simulink model "sim_SIL_code_algorithm"  (R2023a)
settings: Solver=FixedStepAuto  StartTime=0.0  StopTime=Inf  FixedStep=0.01  RelTol=1e-3
model workspace (MAT data in the model file):
  Fe = 0.02
  J = 0.01
  Ke = 0.75
  Kt = 0.75
  L = 1.1
  R = 5.2
libraries: sldrtlib x1
settings Model: Creator=Tu  LastModifiedBy=Tu

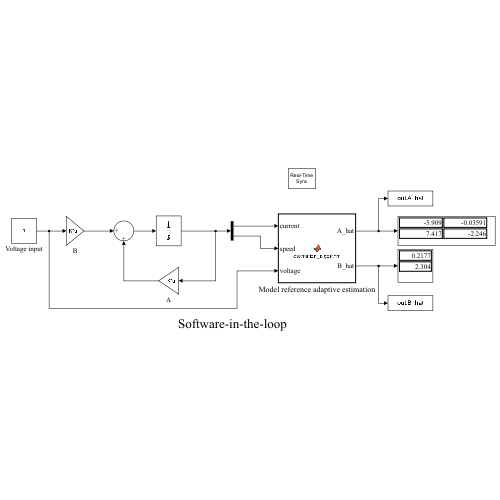
[thumbnail: Simulink's stored preview of the top-level diagram]
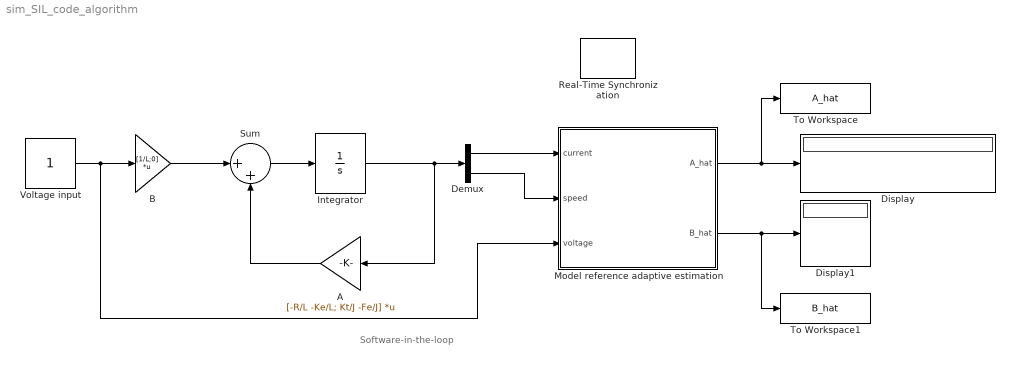
== system sim_SIL_code_algorithm ==
  note: Software-in-the-loop
  A : Gain  Gain=[-R/L -Ke/L; Kt/J -Fe/J]  Multiplication=Matrix(K*u)
  B : Gain  Gain=[1/L;0]  Multiplication=Matrix(K*u)
  Demux : Demux  Outputs=2
  Display : Display
  Display1 : Display
  Integrator : Integrator
  Model reference adaptive estimation : MATLAB Function  TreatAsAtomicUnit=on  SystemSampleTime=0.01
  Real-Time Synchronization : sldrtlib/Real-Time Synchronization  SampleTime=0.01  MaxMissedTicks=100000  ShowMissedTicks=off  YieldWhenWaiting=off
  Sum : Sum  Inputs=|++
  To Workspace : ToWorkspace  VariableName=A_hat  SampleTime=-1
      settings: Save2DSignal=2-D array (concatenate along first dimension)
  To Workspace1 : ToWorkspace  VariableName=B_hat  SampleTime=-1
      settings: Save2DSignal=2-D array (concatenate along first dimension)
  Voltage input : Constant
  wires:
  Sum/1 -> Integrator/1
  Voltage input/1 -> B/1, Model reference adaptive estimation/3(voltage)
  B/1 -> Sum/1
  A/1 -> Sum/2
  Integrator/1 -> A/1, Demux/1
  Demux/2 -> Model reference adaptive estimation/2(speed)
  Demux/1 -> Model reference adaptive estimation/1(current)
  Model reference adaptive estimation/2(B_hat) -> To Workspace1/1, Display1/1
  Model reference adaptive estimation/1(A_hat) -> To Workspace/1, Display/1

== matlab function sim_SIL_code_algorithm/Model reference adaptive estimation ==
  data: current input; speed input; voltage input; A_hat output; B_hat output
function [A_hat, B_hat] = estimation_algorithm(current, speed, voltage)
x = zeros(2,3);
coder.extrinsic('py.sim_SIL_code_algorithm.adaptive_estimation');
x = double(py.sim_SIL_code_algorithm.adaptive_estimation(current, speed, voltage));
A_hat = x(:,1:2);
B_hat = x(:,3);
